simulink model "mavsim_chap6"  (R2016a)
settings: Solver=ode15s  StartTime=0.0  StopTime=10000  RelTol=1e-3
InitFcn:
  | param_chap6
undefined symbols (not defined in the file or in its folder): autopilot, drawAircraft, forces_moments, P, plotmavstatevariables, true_states
libraries: simulink x3
settings Model: Creator=beard  LastModifiedBy=Skyler
settings DataIOCC: LimitDataPoints=on  SaveFormat=Array  SignalLoggingSaveFormat=ModelDataLogs
settings OptimizationCC: ExpressionDepthLimit=2147483647  InitFltsAndDblsToZero=on
settings DebuggingCC: UnderspecifiedInitializationDetection=Classic  MergeDetectMultiDrivingBlocksExec=none  SolverPrmCheckMsg=warning  FcnCallInpInsideContextMsg=UseLocalSettings  StateNameClashWarn=warning
settings HardwareCC: ProdBitPerPointer=32  ProdLargestAtomicFloat=None  ProdIntDivRoundTo=Undefined  ProdEndianess=Unspecified  ProdWordSize=32  ProdHWDeviceType=32-bit Generic
settings ModelReferenceCC: PropagateSignalLabelsOutOfModel=off
settings GRTTargetCC: CombineOutputUpdateFcns=off  GRTInterface=on
settings ConfigComp: CovModelRefEnable=Off  CovSFcnEnable=off

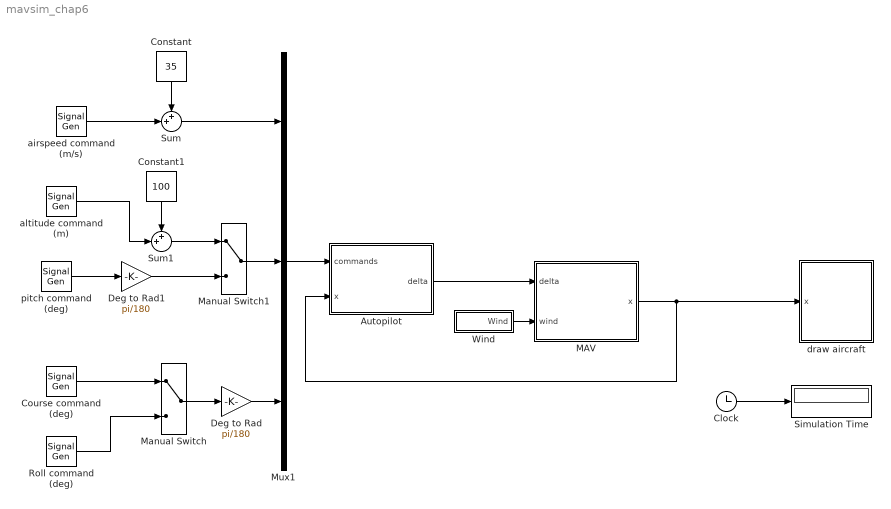
== system mavsim_chap6 ==
  Autopilot : Subsystem
      mask Display: image(imread('kestrel.jpg'))
  Clock : Clock
  Constant : Constant  Value=35
  Constant1 : Constant  Value=100
  Course command (deg) : SignalGenerator  WaveForm=square  Amplitude=30  Frequency=.04
  Deg to Rad : Gain  Gain=pi/180
  Deg to Rad1 : Gain  Gain=pi/180
  MAV : Subsystem
      mask Display: image(imread('batcam.png'))
  Manual Switch : ManualSwitch
  Manual Switch1 : ManualSwitch
  Mux1 : Mux  Inputs=3
  Roll command (deg) : SignalGenerator  WaveForm=square  Amplitude=30  Frequency=.1
  Simulation Time : Display
  Sum : Sum  Inputs=++|
  Sum1 : Sum  Inputs=++|
  Wind : Subsystem
  airspeed command (m/s) : SignalGenerator  WaveForm=square  Amplitude=4  Frequency=.05
  altitude command (m) : SignalGenerator  WaveForm=square  Amplitude=20  Frequency=.03
  draw aircraft : Subsystem
      mask Display: image(imread('tv.jpg'))
  pitch command (deg) : SignalGenerator  WaveForm=square  Amplitude=10  Frequency=.05
  wires:
  Clock/1 -> Simulation Time/1
  Wind/1(Wind) -> MAV/2(wind)
  MAV/1(x) -> draw aircraft/1(x), Autopilot/2(x)
  Autopilot/1(delta) -> MAV/1(delta)
  Mux1/1 -> Autopilot/1(commands)
  Deg to Rad/1 -> Mux1/3
  pitch command (deg)/1 -> Deg to Rad1/1
  Roll command (deg)/1 -> Manual Switch/2
  Manual Switch1/1 -> Mux1/2
  Sum/1 -> Mux1/1
  Constant/1 -> Sum/1
  Sum1/1 -> Manual Switch1/1
  altitude command (m)/1 -> Sum1/2
  Constant1/1 -> Sum1/1
  Course command (deg)/1 -> Manual Switch/1
  Manual Switch/1 -> Deg to Rad/1
  Deg to Rad1/1 -> Manual Switch1/2
  airspeed command (m/s)/1 -> Sum/2

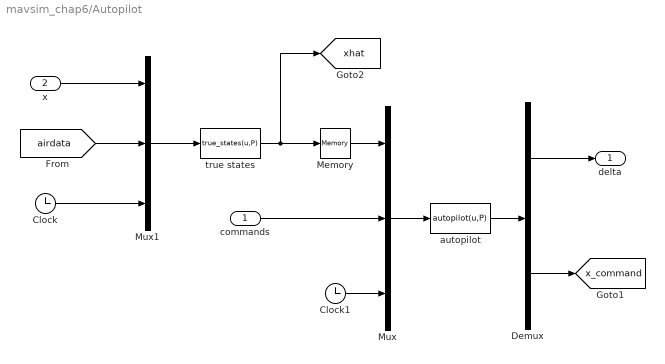
== system mavsim_chap6/Autopilot ==
  commands : Inport
  x : Inport  Port=2
  Clock : Clock
  Clock1 : Clock
  Demux : Demux  Outputs=[4;12]
  Memory : Memory
  Mux : Mux  Inputs=3
  Mux1 : Mux  Inputs=3
  autopilot : MATLABFcn  MATLABFcn=autopilot(u,P)  OutputDimensions=4+12  SampleTime=P.Ts
  true states : MATLABFcn  MATLABFcn=true_states(u,P)  OutputDimensions=19  SampleTime=P.Ts
  delta : Outport
  tag scope: x_command=global, xhat=global
  wires:
  Mux/1 -> autopilot/1
  Clock/1 -> Mux1/3
  autopilot/1 -> Demux/1
  Demux/1 -> delta/1
  Demux/2 -> [x_command]
  commands/1 -> Mux/2
  Mux1/1 -> true states/1
  x/1 -> Mux1/1
  true states/1 -> [xhat], Memory/1
  [airdata] -> Mux1/2
  Memory/1 -> Mux/1
  Clock1/1 -> Mux/3

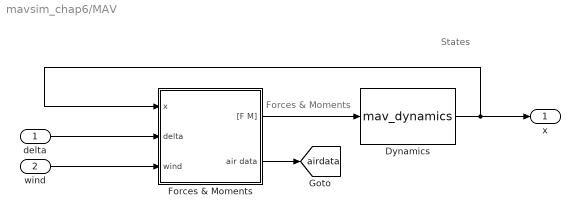
== system mavsim_chap6/MAV ==
  note: Forces & Moments
  note: States
  delta : Inport
  wind : Inport  Port=2
  Dynamics : S-Function  FunctionName=mav_dynamics  Parameters=P  SFunctionDeploymentMode=off  EnableBusSupport=off
  Forces & Moments : Subsystem
  x : Outport
  tag scope: airdata=global
  wires:
  Dynamics/1 -> Forces & Moments/1(x), x/1
  Forces & Moments/1("[F M]") -> Dynamics/1
  Forces & Moments/2(air data) -> [airdata]
  delta/1 -> Forces & Moments/2(delta)
  wind/1 -> Forces & Moments/3(wind)

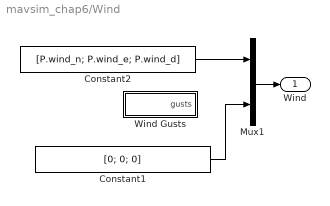
== system mavsim_chap6/Wind ==
  Constant1 : Constant  Value=[0; 0; 0]
  Constant2 : Constant  Value=[P.wind_n; P.wind_e; P.wind_d]
  Mux1 : Mux  Inputs=2
  Wind Gusts : Subsystem
  Wind : Outport
  wires:
  Constant2/1 -> Mux1/1
  Mux1/1 -> Wind/1
  Constant1/1 -> Mux1/2

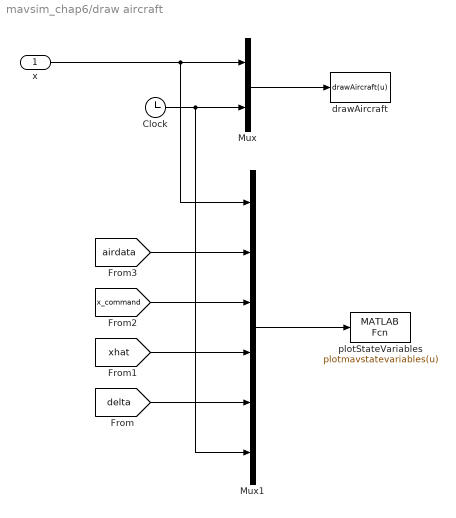
== system mavsim_chap6/draw aircraft ==
  x : Inport
  Clock : Clock
  Mux : Mux  Inputs=2
  Mux1 : Mux  Inputs=6
  drawAircraft : MATLABFcn  MATLABFcn=drawAircraft(u)  OutputDimensions=0  SampleTime=0.1
  plotStateVariables : MATLABFcn  MATLABFcn=plotmavstatevariables(u)  OutputDimensions=0  SampleTime=0.1
  wires:
  Mux/1 -> drawAircraft/1
  x/1 -> Mux/1, Mux1/1
  Clock/1 -> Mux/2, Mux1/6
  Mux1/1 -> plotStateVariables/1
  [xhat] -> Mux1/4
  [x_command] -> Mux1/3
  [delta] -> Mux1/5
  [airdata] -> Mux1/2

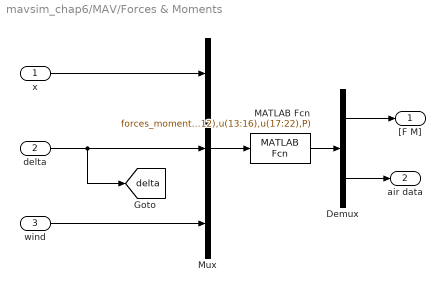
== system mavsim_chap6/MAV/Forces & Moments ==
  x : Inport
  delta : Inport  Port=2
  wind : Inport  Port=3
  Demux : Demux  Outputs=[6;6]
  MATLAB Fcn : MATLABFcn  MATLABFcn=forces_moments(u(1:12),u(13:16),u(17:22),P)  OutputDimensions=12
  Mux : Mux  Inputs=3
  "[F M]" : Outport
  air data : Outport  Port=2
  tag scope: delta=global
  wires:
  Demux/2 -> air data/1
  Mux/1 -> MATLAB Fcn/1
  Demux/1 -> "[F M]"/1
  MATLAB Fcn/1 -> Demux/1
  wind/1 -> Mux/3
  delta/1 -> Mux/2, [delta]
  x/1 -> Mux/1

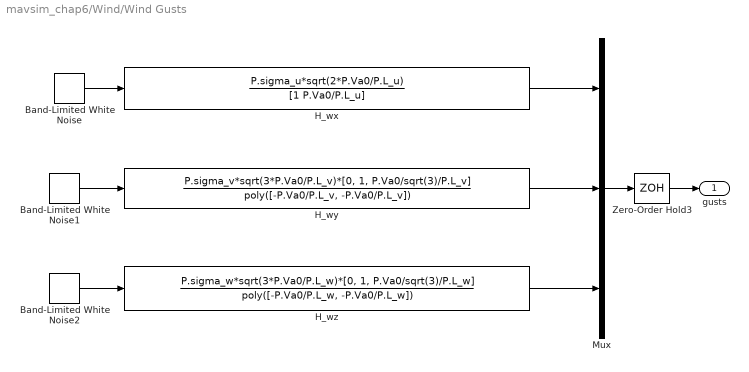
== system mavsim_chap6/Wind/Wind Gusts ==
  Band-Limited White Noise : simulink/Sources/Band-Limited White Noise  Cov=[1]  Ts=P.Ts  seed=[23341]
  Band-Limited White Noise1 : simulink/Sources/Band-Limited White Noise  Cov=[1]  Ts=P.Ts  seed=[23341]
  Band-Limited White Noise2 : simulink/Sources/Band-Limited White Noise  Cov=[1]  Ts=P.Ts  seed=[23341]
  H_wx : TransferFcn  Numerator=P.sigma_u*sqrt(2*P.Va0/P.L_u)  Denominator=[1 P.Va0/P.L_u]
  H_wy : TransferFcn  Numerator=P.sigma_v*sqrt(3*P.Va0/P.L_v)*[0, 1, P.Va0/sqrt(3)/P.L_v]  Denominator=poly([-P.Va0/P.L_v, -P.Va0/P.L_v])
  H_wz : TransferFcn  Numerator=P.sigma_w*sqrt(3*P.Va0/P.L_w)*[0, 1, P.Va0/sqrt(3)/P.L_w]  Denominator=poly([-P.Va0/P.L_w, -P.Va0/P.L_w])
  Mux : Mux  Inputs=3
  Zero-Order Hold3 : ZeroOrderHold  SampleTime=P.Ts
  gusts : Outport
  wires:
  H_wx/1 -> Mux/1
  Band-Limited White Noise/1 -> H_wx/1
  H_wy/1 -> Mux/2
  Band-Limited White Noise1/1 -> H_wy/1
  H_wz/1 -> Mux/3
  Band-Limited White Noise2/1 -> H_wz/1
  Mux/1 -> Zero-Order Hold3/1
  Zero-Order Hold3/1 -> gusts/1
